simulink model "lab3_linear"  (R2019b)
settings: Solver=VariableStepAuto  StartTime=0.0  StopTime=10.0  RelTol=10e-10  AbsTol=10e-10
values from neighbouring files (symbols this model uses):
  A = subs(jacobian(f,x),[x;u],[x_bar;u_bar])    [lab3.m]
  B = subs(jacobian(f,u),[x;u],[x_bar;u_bar])    [lab3.m]
  K = K_LQR2    [lab3.m]
  x0 = 2*[0; 0; pi/24; 0]    [lab3.m]
settings Model: Creator=Alfred  LastModifiedBy=Alfred

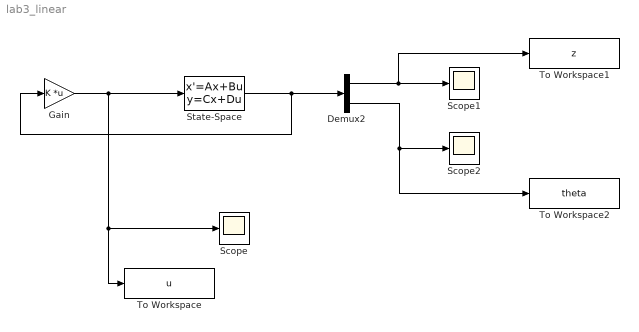
== system lab3_linear ==
  Demux2 : Demux  Outputs=2
  Gain : Gain  Gain=K  Multiplication=Matrix(K*u)
  Scope : Scope
      settings: AttributesFormatString=motor voltage
  Scope1 : Scope
      settings: AttributesFormatString=cart pos
  Scope2 : Scope
      settings: AttributesFormatString=pend angles
  State-Space : StateSpace  A=double(A)  B=double(B)  C=eye(4)  D=zeros(4,1)  InitialCondition=x0
  To Workspace : ToWorkspace  VariableName=u  SaveFormat=Timeseries  SampleTime=-1
  To Workspace1 : ToWorkspace  VariableName=z  SaveFormat=Timeseries  SampleTime=-1
  To Workspace2 : ToWorkspace  VariableName=theta  SaveFormat=Timeseries  SampleTime=-1
  wires:
  State-Space/1 -> Gain/1, Demux2/1
  Demux2/1 -> To Workspace1/1, Scope1/1
  Demux2/2 -> To Workspace2/1, Scope2/1
  Gain/1 -> State-Space/1, To Workspace/1, Scope/1
